simulink model "control_nodos_final_feed"  (R2019a)
settings: Solver=VariableStepAuto  StartTime=0.0  StopTime=600  RelTol=1e-3
values from neighbouring files (symbols this model uses):
  a = -2.0000e-01    (= -0.2)    [programa_nodos.m]
  b = -1.6000e-02    (= -0.016)    [programa_nodos.m]
  c = -6.4000e-04    (= -0.00064)    [programa_nodos.m]
  d = -1.2800e-05    (= -1.28e-05)    [programa_nodos.m]
  e = -1.0240e-07    (= -1.024e-07)    [programa_nodos.m]
  g1 = 2.5000e-02    (= 0.025)    [programa_nodos.m]
  g2 = 1.0000e+00    (= 1)    [programa_nodos.m]
  h = 1.0000e+00    (= 1)    [programa_nodos.m]
  hdis = hdis'    [programa_nodos.m]
  i = 1.0000e+00    (= 1)    [programa_nodos.m]
  j = 1.0000e+00    (= 1)    [programa_nodos.m]
  k = -2.5000e-01    (= -0.25)    [programa_nodos.m]
  l = -3.3141e+00    (= -3.3141)    [programa_nodos.m]
  m = -4.3146e+00    (= -4.3146)    [programa_nodos.m]
  n = 1.0000e+00    (= 1)    [programa_nodos.m]
  o = 1.0000e+00    (= 1)    [programa_nodos.m]
  s = 1.3156e+02    (= 131.56)    [programa_nodos.m]
  tm = 0.5    [programa_nodos.m]
  v = 1.2563e+00    (= 1.2563)    [programa_nodos.m]
  z0 = 0.5    [programa_nodos.m]
  z1 = 0.00000001    (= 1e-08)    [programa_nodos.m]
  z2 = 0.00000001    (= 1e-08)    [programa_nodos.m]
  z3 = 0.00000001    (= 1e-08)    [programa_nodos.m]
  z4 = 0.00000001    (= 1e-08)    [programa_nodos.m]
  z5 = 0.00000001    (= 1e-08)    [programa_nodos.m]
  z6 = 0.00000001    (= 1e-08)    [programa_nodos.m]
  z7 = 0.00000001    (= 1e-08)    [programa_nodos.m]
undefined symbols (not defined in the file or in its folder): A2, adis, B2, bdis, C2, cdis
libraries: simulink x1
settings Model: Creator=Alejoxbg  LastModifiedBy=Alejoxbg

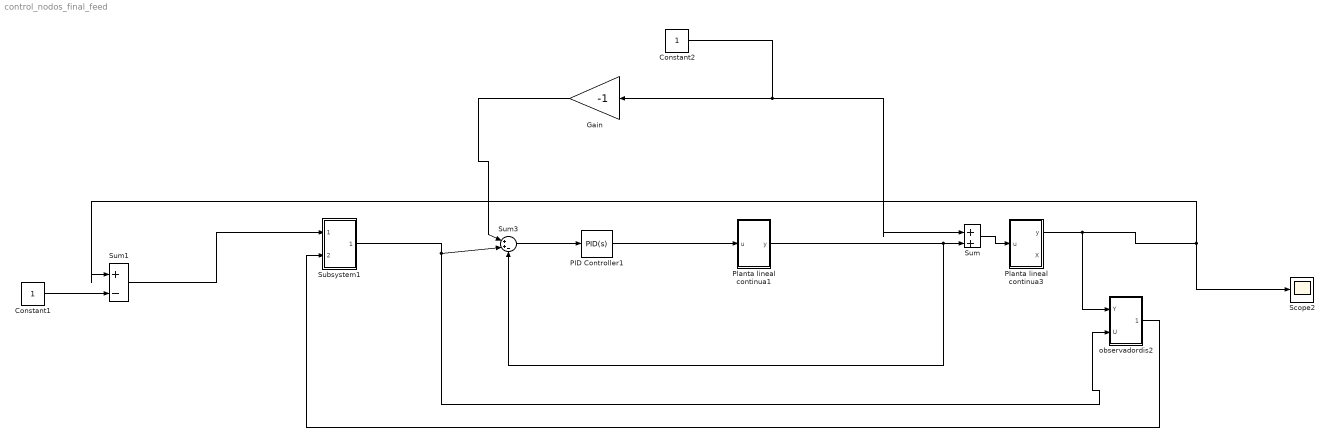
== system control_nodos_final_feed ==
  Constant1 : Constant
  Constant2 : Constant
  Gain : Gain  Gain=-1
  PID Controller1 : simulink/Continuous/PID Controller  Controller=PID  Form=Parallel  TimeDomain=Continuous-time  SampleTime=-1  IntegratorMethod=Forward Euler  FilterMethod=Forward Euler  ControllerParametersSource=internal  P=12.1148539818802  I=1.25631014904339  D=27.6845650272969  UseFilter=on  N=4.3146205312046  TunerSelectOption=Transfer Function Based (PID Tuner App)  InitialConditionSource=internal  InitialConditionForIntegrator=0  InitialConditionForFilter=0  DifferentiatorICPrevScaledInput=0  ExternalReset=none  TrackingMode=off  Kt=1  LimitOutput=off  UpperSaturationLimit=inf  LowerSaturationLimit=-inf  LinearizeAsGain=on  AntiWindupMode=none  Kb=1  POutMin=[]  POutMax=[]  IOutMin=[]  IOutMax=[]  DOutMin=[]  DOutMax=[]  NOutMin=[]  NOutMax=[]  SumOutMin=[]  SumOutMax=[]  SaturationOutMin=[]  SaturationOutMax=[]  PParamMin=[]  PParamMax=[]  IParamMin=[]  IParamMax=[]  DParamMin=[]  DParamMax=[]  NParamMin=[]  NParamMax=[]  KbParamMin=[]  KbParamMax=[]  KtParamMin=[]  KtParamMax=[]  KbOutMin=[]  KbOutMax=[]  KtOutMin=[]  KtOutMax=[]  IntegratorOutMin=[]  IntegratorOutMax=[]  FilterOutMin=[]  FilterOutMax=[]  SumI1OutMin=[]  SumI1OutMax=[]  SumI2OutMin=[]  SumI2OutMax=[]  SumI3OutMin=[]  SumI3OutMax=[]  SumI4OutMin=[]  SumI4OutMax=[]  SumDOutMin=[]  SumDOutMax=[]  DifferentiatorOutMin=[]  DifferentiatorOutMax=[]  FilterDiffOutCoefMin=[]  FilterDiffOutCoefMax=[]  ReciprocalOutMin=[]  ReciprocalOutMax=[]  SumDenOutMin=[]  SumDenOutMax=[]  SumNumOutMin=[]  SumNumOutMax=[]  DivideOutMin=[]  DivideOutMax=[]  IntegratorContinuousStateAttributes=''  IntegratorStateMustResolveToSignalObject=off  IntegratorRTWStateStorageClass=Auto  FilterContinuousStateAttributes=''  FilterStateMustResolveToSignalObject=off  FilterRTWStateStorageClass=Auto  ParallelPVariant=InternalParameters  IdealPVariant=Disabled  IVariant=InternalParameters  DVariant=InternalParameters  IntegratorVariant=Continuous  SatVariant=Disabled  AWVariant=Passthrough  PCopyVariant=Disabled  TRVariant=Disabled  FdbkBlocksVariant=Forward  IdealPFdbkVariant=Disabled  SatFdbkVariant=Disabled  DerivativeFilterVariant=ContFilter  NVariant=InternalParameters  NCopyVariant=Disabled  FilterICVariant=InternalICsFilter  IntegratorICVariant=InternalICs  ExternalResetVariant=Disabled  TRSumVariant=Passthrough  SumFdbkVariant=Disabled  SumVariant=Sum_PID
  Planta lineal continua1 : Subsystem
  Planta lineal continua3 : Subsystem
  Scope2 : Scope
  Subsystem1 : Subsystem
  Sum : Sum  Inputs=|++
  Sum1 : Sum  Inputs=|+-
  Sum3 : Sum  Inputs=|++-
  observadordis2 : Subsystem
  wires:
  Subsystem1/1(Out1) -> observadordis2/2(U), Sum3/2
  observadordis2/1(xgorro) -> Subsystem1/2(In6)
  Planta lineal continua3/1(y) -> observadordis2/1(Y), Sum1/1, Scope2/1
  Constant1/1 -> Sum1/2
  Sum1/1 -> Subsystem1/1(In5)
  Gain/1 -> Sum3/1
  Planta lineal continua1/1(y) -> Sum/2, Sum3/3
  Sum/1 -> Planta lineal continua3/1(u)
  Sum3/1 -> PID Controller1/1
  Constant2/1 -> Sum/1, Gain/1
  PID Controller1/1 -> Planta lineal continua1/1(u)

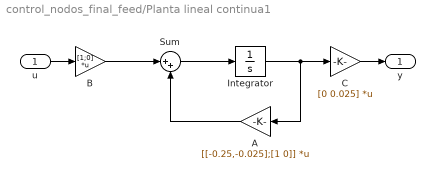
== system control_nodos_final_feed/Planta lineal continua1 ==
  u : Inport
  A : Gain  Gain=[[-0.25,-0.025];[1 0]]  Multiplication=Matrix(K*u) (u vector)
  B : Gain  Gain=[1;0]  Multiplication=Matrix(K*u) (u vector)
  C : Gain  Gain=[0 0.025]  Multiplication=Matrix(K*u) (u vector)
  Integrator : Integrator
  Sum : Sum  Inputs=|++
  y : Outport
  wires:
  C/1 -> y/1
  u/1 -> B/1
  Integrator/1 -> A/1, C/1
  A/1 -> Sum/2
  Sum/1 -> Integrator/1
  B/1 -> Sum/1

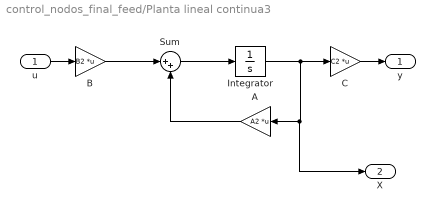
== system control_nodos_final_feed/Planta lineal continua3 ==
  u : Inport
  A : Gain  Gain=A2  Multiplication=Matrix(K*u) (u vector)
  B : Gain  Gain=B2  Multiplication=Matrix(K*u) (u vector)
  C : Gain  Gain=C2  Multiplication=Matrix(K*u) (u vector)
  Integrator : Integrator
  Sum : Sum  Inputs=|++
  y : Outport
  X : Outport  Port=2
  wires:
  C/1 -> y/1
  u/1 -> B/1
  Integrator/1 -> X/1, A/1, C/1
  A/1 -> Sum/2
  Sum/1 -> Integrator/1
  B/1 -> Sum/1

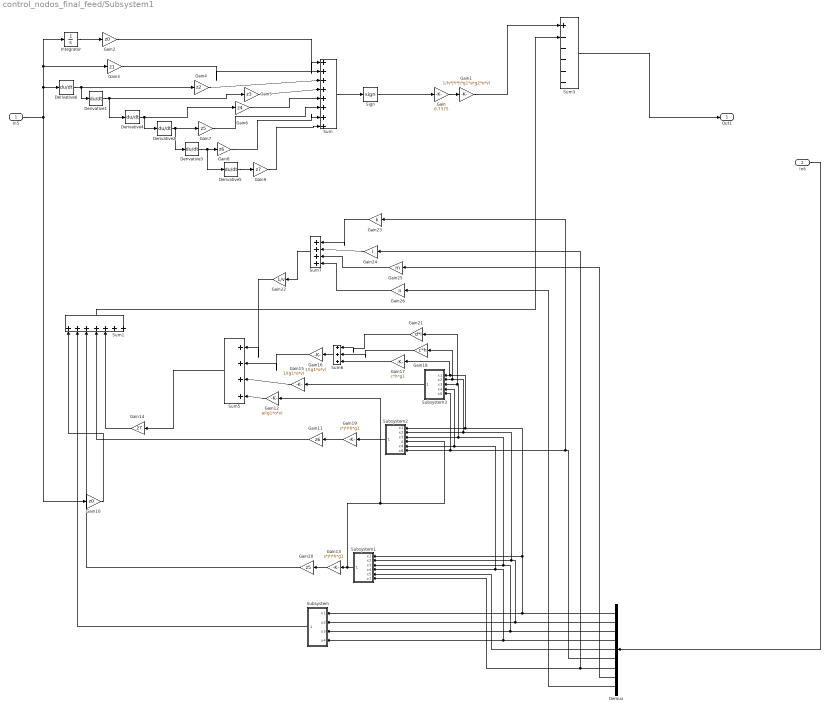
== system control_nodos_final_feed/Subsystem1 ==
  In5 : Inport
  In6 : Inport  Port=2
  Demux : Demux  Outputs=9
  Derivative{1..6} (6 alike) : Derivative
  Gain : Gain  Gain=0.7375
  Gain1 : Gain  Gain=1/(s*j*i*h*g1*a*g2*o*v)
  Gain10 : Gain  Gain=z0
  Gain11 : Gain  Gain=z6
  Gain12 : Gain  Gain=a/(g1*o*v)
  Gain13 : Gain  Gain=s*j*i*h*g1
  Gain14 : Gain  Gain=z7
  Gain15 : Gain  Gain=1/(g1*o*v)
  Gain16 : Gain  Gain=1/(g1*o*v)
  Gain17 : Gain  Gain=c*h*g1
  Gain18 : Gain  Gain=c*h
  Gain19 : Gain  Gain=s*j*i*h*g1
  Gain2 : Gain  Gain=z0
  Gain20 : Gain  Gain=z5
  Gain21 : Gain  Gain=d*i
  Gain22 : Gain  Gain=1/v
  Gain23 : Gain  Gain=k
  Gain24 : Gain  Gain=l
  Gain25 : Gain  Gain=m
  Gain26 : Gain  Gain=n
  Gain3 : Gain  Gain=z1
  Gain4 : Gain  Gain=z2
  Gain5 : Gain  Gain=z3
  Gain6 : Gain  Gain=z4
  Gain7 : Gain  Gain=z5
  Gain8 : Gain  Gain=z6
  Gain9 : Gain  Gain=z7
  Integrator : Integrator
  Sign : Signum  ZeroCross=off
  Subsystem : Subsystem
  Subsystem1 : Subsystem
  Subsystem2 : Subsystem
  Subsystem3 : Subsystem
  Sum : Sum  Inputs=|++++++++
  Sum1 : Sum  Inputs=|+++++++
  Sum3 : Sum  Inputs=|+-----
  Sum5 : Sum  Inputs=|++++
  Sum6 : Sum  Inputs=|+++
  Sum7 : Sum  Inputs=|++++
  Out1 : Outport
  wires:
  Sum/1 -> Sign/1
  Sum6/1 -> Gain16/1
  Subsystem1/1(Out1) -> Gain12/1, Subsystem2/4("sum1 "), Gain13/1
  Demux/3 -> Subsystem/3("x3 "), Subsystem1/3("x3 "), Gain21/1, Subsystem3/3("x3 "), Subsystem2/3("x3 ")
  Sum1/1 -> Sum3/2
  Demux/2 -> Subsystem/2("x2 "), Subsystem1/2("x2 "), Gain18/1, Subsystem3/2("x2 "), Subsystem2/2("x2 ")
  In5/1 -> Derivative6/1, Gain3/1, Integrator/1, Gain10/1
  Gain15/1 -> Sum5/3
  Demux/4 -> Subsystem/4("x4 "), Subsystem1/4("x4 "), Subsystem3/4("x4 "), Subsystem2/5("x4 ")
  Gain21/1 -> Sum6/1
  Gain17/1 -> Sum6/3
  Demux/1 -> Subsystem/1("x1 "), Subsystem1/1("x1 "), Gain17/1, Subsystem3/1("x1 "), Subsystem2/1("x1 ")
  Demux/6 -> Gain23/1, Subsystem3/5("x6 "), Subsystem2/6("x6 ")
  Gain10/1 -> Sum1/1
  Subsystem2/1(Out1) -> Gain19/1
  Demux/7 -> Gain24/1, Subsystem1/6("x7 ")
  Demux/5 -> Subsystem1/5("x5 ")
  Gain13/1 -> Gain20/1
  Gain12/1 -> Sum5/4
  Gain4/1 -> Sum/3
  Sum5/1 -> Gain14/1
  Demux/8 -> Gain25/1
  Gain18/1 -> Sum6/2
  Derivative1/1 -> Derivative4/1, Gain5/1
  Gain22/1 -> Sum5/1
  Gain23/1 -> Sum7/1
  Gain25/1 -> Sum7/3
  Gain19/1 -> Gain11/1
  Gain24/1 -> Sum7/2
  Gain3/1 -> Sum/2
  Demux/9 -> Gain26/1
  Gain11/1 -> Sum1/4
  Gain26/1 -> Sum7/4
  Gain16/1 -> Sum5/2
  Subsystem3/1(Out1) -> Gain15/1
  Subsystem/1(Out1) -> Sum1/2
  Gain/1 -> Gain1/1
  Derivative3/1 -> Derivative5/1, Gain8/1
  Derivative4/1 -> Derivative2/1, Gain6/1
  Derivative5/1 -> Gain9/1
  Sign/1 -> Gain/1
  Derivative6/1 -> Derivative1/1, Gain4/1
  Gain7/1 -> Sum/6
  Integrator/1 -> Gain2/1
  Gain20/1 -> Sum1/3
  Gain2/1 -> Sum/1
  Derivative2/1 -> Derivative3/1, Gain7/1
  Gain5/1 -> Sum/4
  Gain6/1 -> Sum/5
  Gain1/1 -> Sum3/1
  Gain9/1 -> Sum/8
  Gain8/1 -> Sum/7
  Sum7/1 -> Gain22/1
  Gain14/1 -> Sum1/5
  Sum3/1 -> Out1/1
  In6/1 -> Demux/1

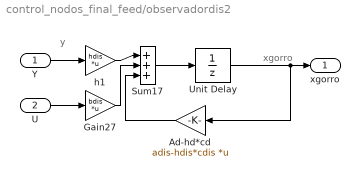
== system control_nodos_final_feed/observadordis2 ==
  note: xgorro
  note: y
  Y : Inport
  U : Inport  Port=2
  Ad-hd*cd : Gain  Gain=adis-hdis*cdis  Multiplication=Matrix(K*u) (u vector)  SampleTime=tm
  Gain27 : Gain  Gain=bdis  Multiplication=Matrix(K*u) (u vector)  SampleTime=tm
  Sum17 : Sum  Inputs=|+++
  Unit Delay : UnitDelay  SampleTime=tm  HasFrameUpgradeWarning=on
  h1 : Gain  Gain=hdis  Multiplication=Matrix(K*u) (u vector)  SampleTime=tm
  xgorro : Outport
  wires:
  Sum17/1 -> Unit Delay/1
  h1/1 -> Sum17/1
  Unit Delay/1 -> Ad-hd*cd/1, xgorro/1
  Ad-hd*cd/1 -> Sum17/3
  Gain27/1 -> Sum17/2
  Y/1 -> h1/1
  U/1 -> Gain27/1

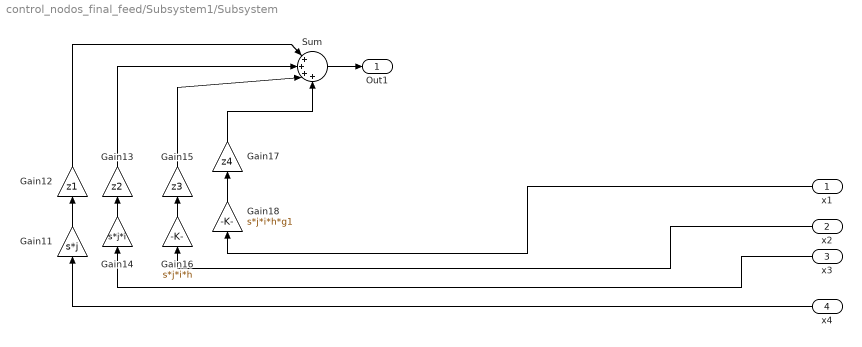
== system control_nodos_final_feed/Subsystem1/Subsystem ==
  "x1 " : Inport
  "x2 " : Inport  Port=2
  "x3 " : Inport  Port=3
  "x4 " : Inport  Port=4
  Gain11 : Gain  Gain=s*j
  Gain12 : Gain  Gain=z1
  Gain13 : Gain  Gain=z2
  Gain14 : Gain  Gain=s*j*i
  Gain15 : Gain  Gain=z3
  Gain16 : Gain  Gain=s*j*i*h
  Gain17 : Gain  Gain=z4
  Gain18 : Gain  Gain=s*j*i*h*g1
  Sum : Sum  Inputs=|++++
  Out1 : Outport
  wires:
  Gain18/1 -> Gain17/1
  Gain11/1 -> Gain12/1
  Gain16/1 -> Gain15/1
  "x3 "/1 -> Gain14/1
  "x1 "/1 -> Gain18/1
  Gain14/1 -> Gain13/1
  "x4 "/1 -> Gain11/1
  "x2 "/1 -> Gain16/1
  Sum/1 -> Out1/1
  Gain17/1 -> Sum/4
  Gain15/1 -> Sum/3
  Gain13/1 -> Sum/2
  Gain12/1 -> Sum/1

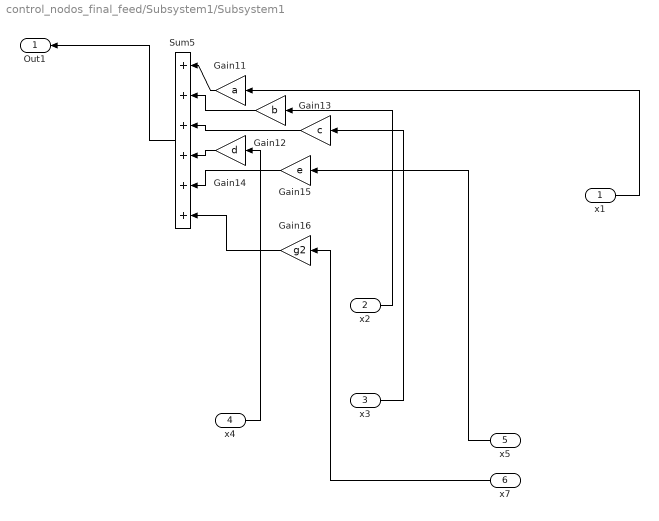
== system control_nodos_final_feed/Subsystem1/Subsystem1 ==
  "x1 " : Inport
  "x2 " : Inport  Port=2
  "x3 " : Inport  Port=3
  "x4 " : Inport  Port=4
  "x5 " : Inport  Port=5
  "x7 " : Inport  Port=6
  Gain11 : Gain  Gain=a
  Gain12 : Gain  Gain=b
  Gain13 : Gain  Gain=c
  Gain14 : Gain  Gain=d
  Gain15 : Gain  Gain=e
  Gain16 : Gain  Gain=g2
  Sum5 : Sum  Inputs=|++++++
  Out1 : Outport
  wires:
  Sum5/1 -> Out1/1
  Gain12/1 -> Sum5/2
  Gain16/1 -> Sum5/6
  Gain13/1 -> Sum5/3
  "x3 "/1 -> Gain13/1
  Gain11/1 -> Sum5/1
  Gain14/1 -> Sum5/4
  Gain15/1 -> Sum5/5
  "x4 "/1 -> Gain14/1
  "x1 "/1 -> Gain11/1
  "x7 "/1 -> Gain16/1
  "x5 "/1 -> Gain15/1
  "x2 "/1 -> Gain12/1

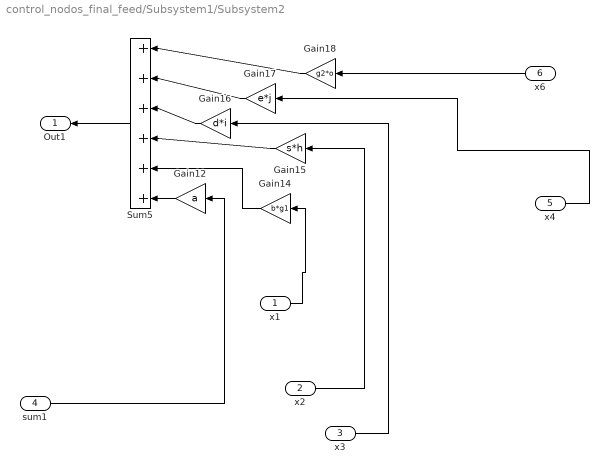
== system control_nodos_final_feed/Subsystem1/Subsystem2 ==
  "x1 " : Inport
  "x2 " : Inport  Port=2
  "x3 " : Inport  Port=3
  "sum1 " : Inport  Port=4
  "x4 " : Inport  Port=5
  "x6 " : Inport  Port=6
  Gain12 : Gain  Gain=a
  Gain14 : Gain  Gain=b*g1
  Gain15 : Gain  Gain=s*h
  Gain16 : Gain  Gain=d*i
  Gain17 : Gain  Gain=e*j
  Gain18 : Gain  Gain=g2*o
  Sum5 : Sum  Inputs=|++++++
  Out1 : Outport
  wires:
  Gain12/1 -> Sum5/6
  Gain15/1 -> Sum5/4
  "x6 "/1 -> Gain18/1
  Gain18/1 -> Sum5/1
  "sum1 "/1 -> Gain12/1
  Gain16/1 -> Sum5/3
  Gain14/1 -> Sum5/5
  Gain17/1 -> Sum5/2
  "x1 "/1 -> Gain14/1
  "x2 "/1 -> Gain15/1
  "x4 "/1 -> Gain17/1
  "x3 "/1 -> Gain16/1
  Sum5/1 -> Out1/1

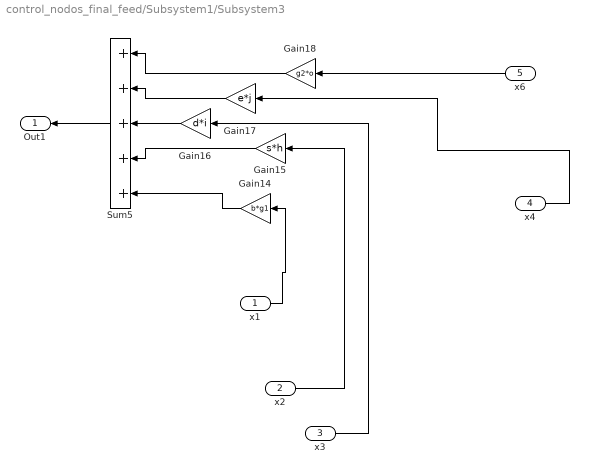
== system control_nodos_final_feed/Subsystem1/Subsystem3 ==
  "x1 " : Inport
  "x2 " : Inport  Port=2
  "x3 " : Inport  Port=3
  "x4 " : Inport  Port=4
  "x6 " : Inport  Port=5
  Gain14 : Gain  Gain=b*g1
  Gain15 : Gain  Gain=s*h
  Gain16 : Gain  Gain=d*i
  Gain17 : Gain  Gain=e*j
  Gain18 : Gain  Gain=g2*o
  Sum5 : Sum  Inputs=|+++++
  Out1 : Outport
  wires:
  Gain15/1 -> Sum5/4
  "x6 "/1 -> Gain18/1
  Gain18/1 -> Sum5/1
  Gain16/1 -> Sum5/3
  Gain14/1 -> Sum5/5
  Gain17/1 -> Sum5/2
  "x1 "/1 -> Gain14/1
  "x2 "/1 -> Gain15/1
  "x4 "/1 -> Gain17/1
  "x3 "/1 -> Gain16/1
  Sum5/1 -> Out1/1
